simulink library "its"  (Simulink 8.1)
settings: Solver=ode1  StartTime=0.0  StopTime=Inf  FixedStep=0.001  RelTol=1e-3
PostLoadFcn:
  | , if any(exist('dsrtsu_mdlpostloadfcn', 'file') == [2, 3, 6]), try dsrtsu_mdlpostloadfcn('Execute', bdroot); catch fprintf('Error in PostLoadFcn (dsrtsu_mdlpostloadfcn) for model "%s":\n %s\n', bdroot, lasterr); end, end,
undefined symbols (not defined in the file or in its folder): KACC_ACCStopDistDecelFormula_m, KACC_DecelDistCtrlIntToStopDefault_mps2
libraries: hcu_lib x1
settings Model: DSRTSU_INTERNAL_RTI_VER=450  DSRTSU_INTERNAL_RTI_TYPE=rti1401  Creator=AT015555  LastModifiedBy=AT015555

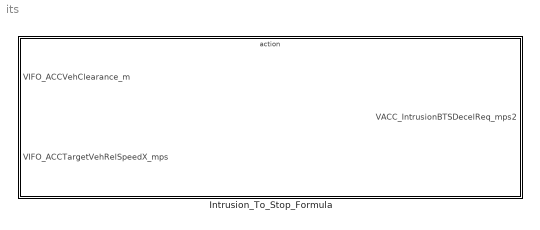
== system its ==
  Intrusion_To_Stop_Formula : Subsystem  TreatAsAtomicUnit=on

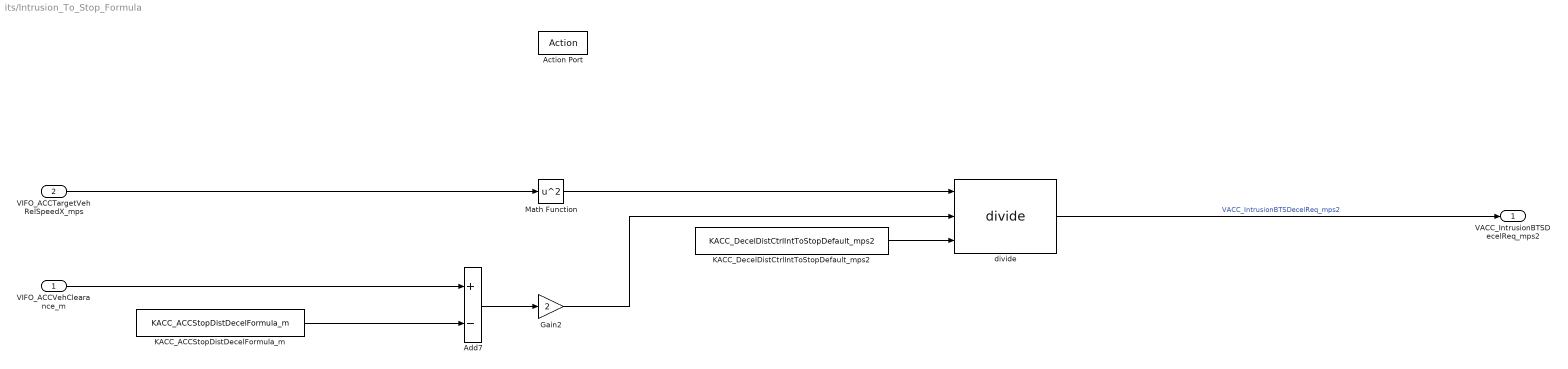
== system its/Intrusion_To_Stop_Formula ==
  VIFO_ACCVehClearance_m : Inport
  VIFO_ACCTargetVehRelSpeedX_mps : Inport  Port=2
  Action Port : ActionPort
  Add7 : Sum  Inputs=+-
  Gain2 : Gain  Gain=2
  KACC_ACCStopDistDecelFormula_m : Constant  Value=KACC_ACCStopDistDecelFormula_m
  KACC_DecelDistCtrlIntToStopDefault_mps2 : Constant  Value=KACC_DecelDistCtrlIntToStopDefault_mps2
  Math Function : Math  Operator=square  SaturateOnIntegerOverflow=on
  divide : hcu_lib/divide
  VACC_IntrusionBTSDecelReq_mps2 : Outport
  wires:
  KACC_ACCStopDistDecelFormula_m/1 -> Add7/2
  KACC_DecelDistCtrlIntToStopDefault_mps2/1 -> divide/3
  Gain2/1 -> divide/2
  Add7/1 -> Gain2/1
  Math Function/1 -> divide/1
  VIFO_ACCTargetVehRelSpeedX_mps/1 -> Math Function/1
  VIFO_ACCVehClearance_m/1 -> Add7/1
  divide/1 -> VACC_IntrusionBTSDecelReq_mps2/1  "VACC_IntrusionBTSDecelReq_mps2"
